simulink model "pendulum_simulation"  (R2023b)
settings: Solver=VariableStepAuto  StartTime=0.0  StopTime=10.0  RelTol=1e-3
settings Model: Creator=frede  LastModifiedBy=frede
settings DataIOCC: Refine=10

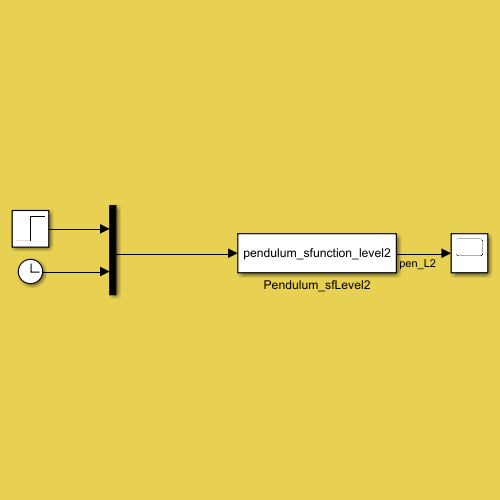
[thumbnail: Simulink's stored preview of the top-level diagram]
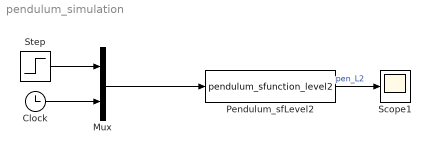
== system pendulum_simulation ==
  Clock : Clock
  Mux : Mux  Inputs=2
  Pendulum_sfLevel2 : M-S-Function  FunctionName=pendulum_sfunction_level2  Parameters=pi/4 0
  Scope1 : Scope
  Step : Step  After=1e-2  SampleTime=0
  wires:
  Pendulum_sfLevel2/1 -> Scope1/1  "pen_L2"
  Clock/1 -> Mux/2
  Mux/1 -> Pendulum_sfLevel2/1
  Step/1 -> Mux/1
